simulink model "Ejercicio6_27_03_17"  (R2013a)
settings: Solver=ode45  StartTime=0.0  StopTime=0.1  RelTol=1e-3
libraries: powerlib x9
settings Model: Creator=Miguel  LastModifiedBy=Miguel

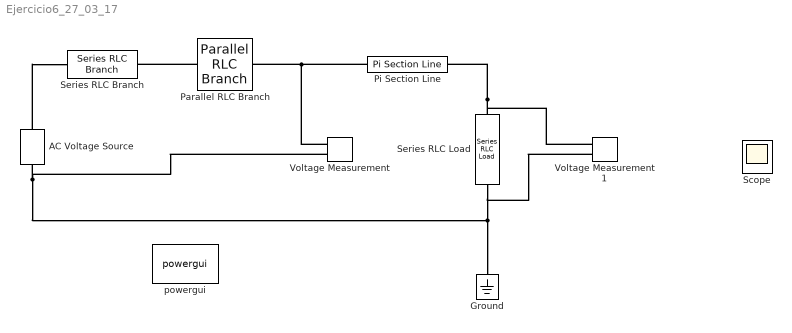
== system Ejercicio6_27_03_17 ==
  AC Voltage Source : powerlib/Electrical Sources/AC Voltage Source  Amplitude=sqrt(2)*424.4e3  Phase=0  Frequency=60  SampleTime=0  Measurements=None
  Ground : powerlib/Elements/Ground  LConnTagsString=a
  Parallel RLC Branch : powerlib/Elements/Parallel RLC Branch  LConnTagsString=a  RConnTagsString=__new0  BranchType=RLC  Resistance=180.1  Inductance=26.525e-3  SetiL0=off  InitialCurrent=0  Capacitance=117.84e-6  Setx0=off  InitialVoltage=0  Measurements=None
  Pi Section Line : powerlib/Elements/Pi Section Line  LConnTagsString=__new0  RConnTagsString=__new0  Frequency=60  Resistance=0.011  Inductance=0.8674e-3  Capacitance=13.41e-9  Length=300  PiSections=1  Measurements=None
      settings: AttributesFormatString=\n
  Scope : Scope  NumInputPorts=2
      settings: ShowLegends=on  YMin=-5~-5  YMax=5~5
  Series RLC Branch : powerlib/Elements/Series RLC Branch  LConnTagsString=__new0  RConnTagsString=__new0  BranchType=R  Resistance=2  Inductance=1e-3  SetiL0=off  InitialCurrent=0  Capacitance=1e-6  Setx0=off  InitialVoltage=0  Measurements=None
  Series RLC Load : powerlib/Elements/Series RLC Load  LConnTagsString=a  RConnTagsString=__new0  NominalVoltage=424.4e3  NominalFrequency=60  ActivePower=110e6/300  InductivePower=110e6  CapacitivePower=0  Setx0=off  InitialVoltage=0  SetiL0=off  InitialCurrent=0  Measurements=None
  Voltage Measurement : powerlib/Measurements/Voltage Measurement  PhasorSimulation=on  OutputType=Complex  PSBequivalent=0
  Voltage Measurement1 : powerlib/Measurements/Voltage Measurement  PhasorSimulation=on  OutputType=Complex  PSBequivalent=0
  powergui : powerlib/powergui  Priority=1  SimulationMode=Phasor  SolverType=Tustin  SampleTime=50e-6  frequency=60  SPID=off  DisableSnubberDevices=off  DisableRonSwitches=off  DisableVfSwitches=off  SwTol=0  Interpol=off  DisplayEquations=off  frequencyindice=60  Pbase=100e6  ErrMax=1e-4  Iterations=50  UnitsV=kV  UnitsW=MW  FunctionMessages=off  echomessages=off  HookPort=off  EnableUseOfTLC=off  x0status=blocks  RestoreLinks=warning  ResistiveCurrentMeasurement=off  Frange=[0:2:500]  Ylog=off  Xlog=on  ShowGrid=off  save=off  variable=ZData  ZoomFFT=off  StartTime=0.0  cycles=1  DisplayStyle=1  fundamental=60  FreqAxis=off  MaxFrequency=1000  frequencyindicesteady=1  RmsSteady=1  display=off  Ts=0  methode=off
  connections:
  AC Voltage Source/RConn1 -- Series RLC Branch/LConn1
  Parallel RLC Branch/LConn1 -- Series RLC Branch/RConn1
  Series RLC Load/LConn1 -- Pi Section Line/RConn1 -- Voltage Measurement1/LConn1
  AC Voltage Source/LConn1 -- Ground/LConn1 -- Voltage Measurement1/LConn2 -- Series RLC Load/RConn1 -- Voltage Measurement/LConn2
  Pi Section Line/LConn1 -- Voltage Measurement/LConn1 -- Parallel RLC Branch/RConn1
